simulink model "discretefilter_ref_test"  (Simulink 8.4)
settings: Solver=ode45  StartTime=0.0  StopTime=10.0  RelTol=1e-3
settings Model: Creator=arnaud  LastModifiedBy=arnaud
settings DataIOCC: SaveFormat=Structure  SignalLoggingSaveFormat=Dataset
settings OptimizationCC: ExpressionDepthLimit=128
settings DebuggingCC: UnderspecifiedInitializationDetection=Simplified  MergeDetectMultiDrivingBlocksExec=error  FcnCallInpInsideContextMsg=EnableAllAsError  StateNameClashWarn=none
settings GRTTargetCC: CombineOutputUpdateFcns=on  GRTInterface=off

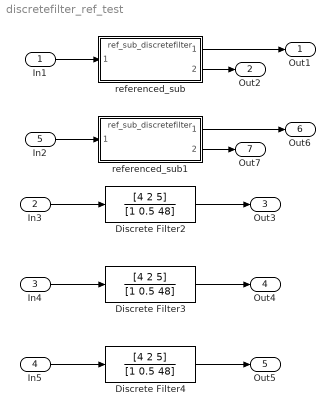
== system discretefilter_ref_test ==
  In1 : Inport
  In3 : Inport  Port=2  PortDimensions=3
  In4 : Inport  Port=3  PortDimensions=[2 3]
  In5 : Inport  Port=4  PortDimensions=[1 3]
  In2 : Inport  Port=5
  Discrete Filter2 : DiscreteFilter  Numerator=[4 2 5]  Denominator=[1 0.5 48]  InitialStates=[1 0.9]  SampleTime=1
  Discrete Filter3 : DiscreteFilter  Numerator=[4 2 5]  Denominator=[1 0.5 48]  InitialStates=[1 0.9]  SampleTime=1
  Discrete Filter4 : DiscreteFilter  Numerator=[4 2 5]  Denominator=[1 0.5 48]  InitialStates=[1 0.9]  SampleTime=1
  referenced_sub : ModelReference  ModelNameDialog=ref_sub_discretefilter.slx  SimulationMode=Normal  ModelReferenceVersion=1.85  CopyOfModelName=ref_sub_discretefilter.slx  DefaultDataLogging=on
  referenced_sub1 : ModelReference  ModelNameDialog=ref_sub_discretefilter.slx  SimulationMode=Normal  ModelReferenceVersion=1.85  CopyOfModelName=ref_sub_discretefilter.slx  DefaultDataLogging=on
  Out1 : Outport
  Out2 : Outport  Port=2
  Out3 : Outport  Port=3
  Out4 : Outport  Port=4
  Out5 : Outport  Port=5
  Out6 : Outport  Port=6
  Out7 : Outport  Port=7
  wires:
  referenced_sub/1 -> Out1/1
  referenced_sub/2 -> Out2/1
  In3/1 -> Discrete Filter2/1
  Discrete Filter2/1 -> Out3/1
  In4/1 -> Discrete Filter3/1
  Discrete Filter3/1 -> Out4/1
  In5/1 -> Discrete Filter4/1
  Discrete Filter4/1 -> Out5/1
  In1/1 -> referenced_sub/1
  referenced_sub1/1 -> Out6/1
  referenced_sub1/2 -> Out7/1
  In2/1 -> referenced_sub1/1
